simulink model "Calculator"  (R2021a)
settings: Solver=FixedStepDiscrete  StartTime=0.0  StopTime=10.0  RelTol=1e-3  EnableMultiTasking=on
libraries: simulink x2
settings Model: Creator=Rana  LastModifiedBy=Rana
settings DataIOCC: ReturnWorkspaceOutputs=off
settings OptimizationCC: DefaultParameterBehavior=Inlined  InlineInvariantSignals=on  EnableMemcpy=off  LifeSpan=1  EfficientTunableParamExpr=on
settings DebuggingCC: UnderspecifiedInitializationDetection=Classic  MergeDetectMultiDrivingBlocksExec=none  SFMachineParentedDataDiag=warning  ArithmeticOperatorsInVariantConditions=warning
settings ModelReferenceCC: PropagateSignalLabelsOutOfModel=off
settings SFSimCC: MATLABDynamicMemAlloc=off  CustomCodeUndefinedFunction=UseInterfaceOnly
settings RTWCC: SystemTargetFile=ert.tlc  GenCodeOnly=on  TemplateMakefile=ert_default_tmf  GenerateReport=on  IncludeHyperlinkInReport=on  LaunchReport=on  GenerateTraceInfo=on  GenerateTraceReport=on  GenerateTraceReportSl=on  GenerateTraceReportSf=on  GenerateTraceReportEml=on
settings CodeAppCC: ForceParamTrailComments=on  IgnoreCustomStorageClasses=off  OperatorAnnotations=on  SimulinkDataObjDesc=on  SFDataObjDesc=on  MATLABFcnDesc=on  InsertBlockDesc=on  StateflowObjectComments=on  MATLABSourceComments=on
settings ERTTargetCC: MultiwordLength=2048  GenerateSampleERTMain=on  InlinedParameterPlacement=NonHierarchical  ERTCustomFileTemplate=example_file_process.tlc

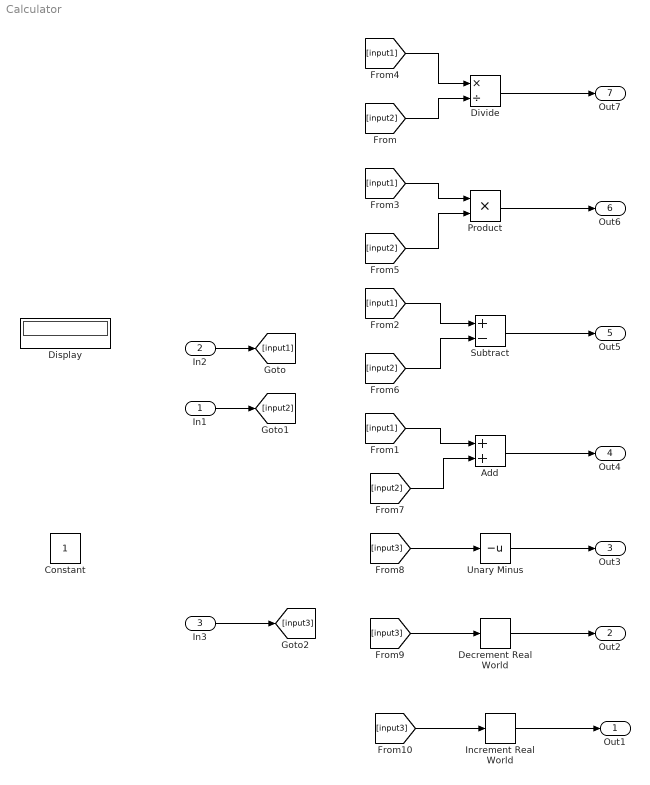
== system Calculator ==
  In1 : Inport
  In2 : Inport  Port=2
  In3 : Inport  Port=3
  Add : Sum
  Constant : Constant
  Decrement Real World : simulink/Additional Math & Discrete/Additional Math: Increment - Decrement/Decrement Real World
      settings: SourceProductBaseCode=SL
  Display : Display
  Divide : Product  Inputs=*/
  Increment Real World : simulink/Additional Math & Discrete/Additional Math: Increment - Decrement/Increment Real World
      settings: SourceProductBaseCode=SL
  Product : Product
  Subtract : Sum  Inputs=+-
  Unary Minus : UnaryMinus
  Out1 : Outport  SignalName=inc
  Out2 : Outport  Port=2  SignalName=dec
  Out3 : Outport  Port=3  SignalName=unary_minus
  Out4 : Outport  Port=4  SignalName=add
  Out5 : Outport  Port=5  SignalName=sub
  Out6 : Outport  Port=6  SignalName=mul
  Out7 : Outport  Port=7  SignalName=div
  wires:
  In2/1 -> [input1]
  [input1] -> Add/1
  [input1] -> Subtract/1
  [input1] -> Product/1
  [input1] -> Divide/1
  In1/1 -> [input2]
  [input2] -> Divide/2
  [input2] -> Product/2
  [input2] -> Subtract/2
  [input2] -> Add/2
  Divide/1 -> Out7/1
  Product/1 -> Out6/1
  Subtract/1 -> Out5/1
  Add/1 -> Out4/1
  Unary Minus/1 -> Out3/1
  Decrement Real World/1 -> Out2/1
  Increment Real World/1 -> Out1/1
  [input3] -> Unary Minus/1
  [input3] -> Decrement Real World/1
  [input3] -> Increment Real World/1
  In3/1 -> [input3]
